simulink model "pendulum_model_PI"  (R2022b)
settings: Solver=VariableStepAuto  StartTime=0.0  StopTime=15  RelTol=1e-3
InitFcn:
  | % LRS TU KL %
  | % By Alen Turnwald %
  | % 09.01.2017 %
  | % clc
  | % close
  | 
  | %% g_q
  | % g_q = [1;0];
  | 
  | 
  | % if ~exist('mp','var')||~exist('mc','var')||~exist('L','var')||~exist('g','var')||~exist('d1','var')||~exist('d2','var')
  | % Model Paramter
  |     % warning(['(Some) Model Parameter are not defined!' ,10, '****  Setting the predefined parameter  ****'])
  |     % N = 2;
  |     % mc = 1.5;
  |     % mp = 0.5;
  |     % g = 9.82;
  |     % L = 1;
  | % Damping factors
  |     % d1 = 1e-2;
  |     % d2 = 1e-2;
  | % end
  | 
  | % if ~exist('x_0','var')
  | % Initial state
  |     % warning(['(Initial state "x_0" not defined or wrongly named!' ,10, '****  Setting x_0 = [0.1; 10 deg; 0; 0]  ****'])
  |     % x_0 = zeros(4,1);
  |     % x_0(1) = 0.1;
  |     % x_0(2) = 10*pi/180;
  | % end
  | 
  | % if ~exist('K_lqr','var')||~exist('Kd_lqr','var')
  | %    warning(['(No controller found!' ,10, '****   Applying a predefined controller  ****'])
  | %    K_lqr = [-14.1421  171.8846  -25.2787   54.7535];
  | % end
undefined symbols (not defined in the file or in its folder): A, B, b_pitching, b_rolling, disturbance, K_d_angle, K_i_pitch, K_p_pitch, period, pulse_width, stall_T, target_angle, x_0
libraries: slpidlib x1
settings Model: Creator=Jake  LastModifiedBy=Jake

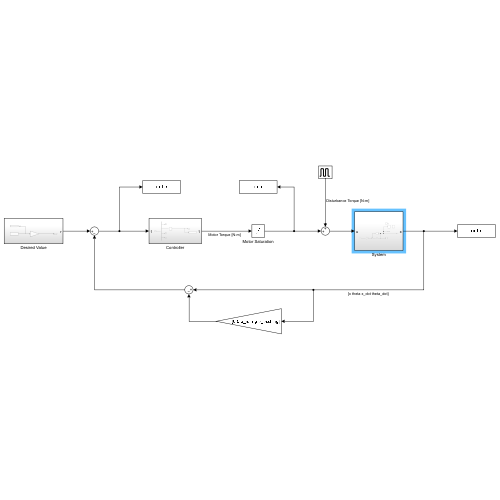
[thumbnail: Simulink's stored preview of the top-level diagram]
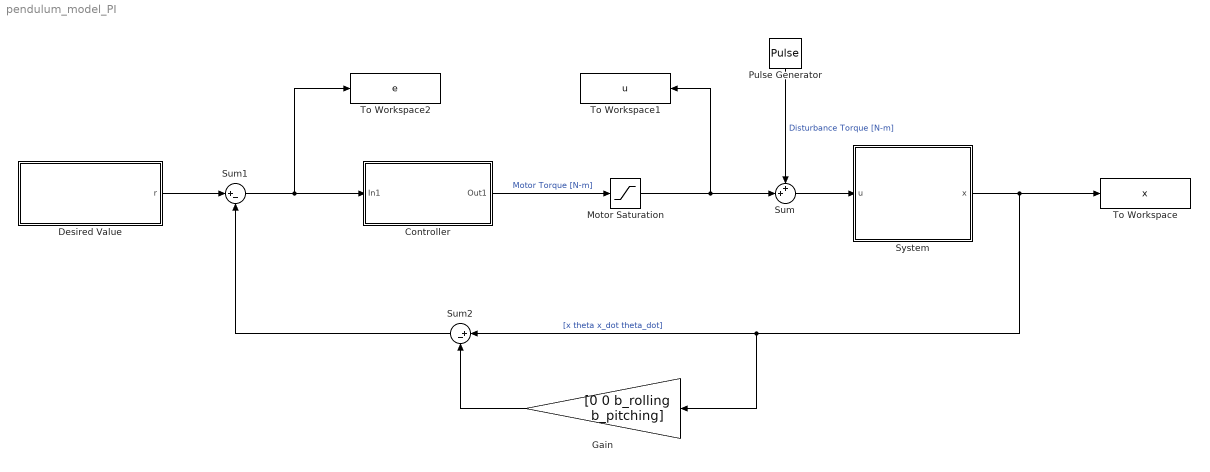
== system pendulum_model_PI ==
  Controller : Subsystem
  Desired Value : Subsystem
  Gain : Gain  Gain=[0 0 b_rolling b_pitching]
  Motor Saturation : Saturate  UpperLimit=stall_T  LowerLimit=-stall_T
  Pulse Generator : DiscretePulseGenerator  PulseType=Time based  Amplitude=disturbance  Period=period  PulseWidth=pulse_width
  Sum : Sum  Inputs=++|
  Sum1 : Sum  Inputs=|+-
  Sum2 : Sum  Inputs=|+-
  System : Subsystem
  To Workspace : ToWorkspace  VariableName=x  SampleTime=-1
  To Workspace1 : ToWorkspace  VariableName=u  SampleTime=-1
  To Workspace2 : ToWorkspace  VariableName=e  SampleTime=-1
  wires:
  Sum/1 -> System/1(u)
  Motor Saturation/1 -> To Workspace1/1, Sum/2
  Pulse Generator/1 -> Sum/1  "Disturbance Torque [N-m]"
  Desired Value/1(r) -> Sum1/1
  Controller/1(Out1) -> Motor Saturation/1  "Motor Torque [N-m]"
  Sum1/1 -> To Workspace2/1, Controller/1(In1)
  System/1(x) -> To Workspace/1, Sum2/1, Gain/1  "[x theta x_dot theta_dot]"
  Sum2/1 -> Sum1/2
  Gain/1 -> Sum2/2

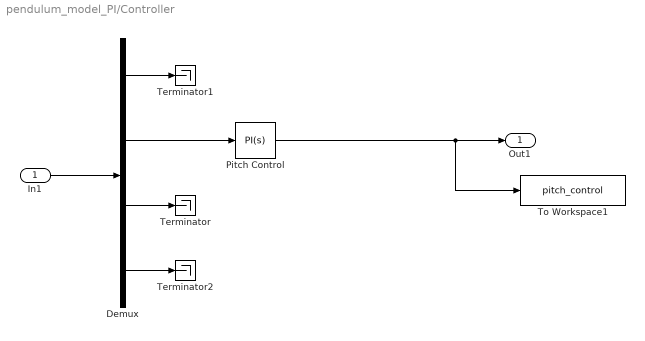
== system pendulum_model_PI/Controller ==
  In1 : Inport
  Demux : Demux
  Pitch Control : slpidlib/PID Controller  Controller=PI  Form=Parallel  TimeDomain=Continuous-time  UseExternalTs=off  SampleTime=-1  IntegratorMethod=Forward Euler  FilterMethod=Forward Euler  ControllerParametersSource=internal  P=K_p_pitch  I=K_i_pitch  UseKiTs=off  D=K_d_angle  N=45  UseFilter=on  TunerSelectOption=Transfer Function Based (PID Tuner App)  InitialConditionSource=internal  InitialConditionForIntegrator=0  InitialConditionForFilter=0  DifferentiatorICPrevScaledInput=0  ExternalReset=none  TrackingMode=off  Kt=1  LimitOutput=off  SatLimitsSource=internal  UpperSaturationLimit=inf  LowerSaturationLimit=-inf  LinearizeAsGain=on  AntiWindupMode=none  Kb=1  LimitIntegrator=off  UpperIntegratorSaturationLimit=inf  LowerIntegratorSaturationLimit=-inf  POutMin=[]  POutMax=[]  IOutMin=[]  IOutMax=[]  DOutMin=[]  DOutMax=[]  NOutMin=[]  NOutMax=[]  SumOutMin=[]  SumOutMax=[]  SaturationOutMin=[]  SaturationOutMax=[]  PParamMin=[]  PParamMax=[]  IParamMin=[]  IParamMax=[]  DParamMin=[]  DParamMax=[]  NParamMin=[]  NParamMax=[]  KbParamMin=[]  KbParamMax=[]  KtParamMin=[]  KtParamMax=[]  KbOutMin=[]  KbOutMax=[]  KtOutMin=[]  KtOutMax=[]  IntegratorOutMin=[]  IntegratorOutMax=[]  FilterOutMin=[]  FilterOutMax=[]  SumI1OutMin=[]  SumI1OutMax=[]  SumI2OutMin=[]  SumI2OutMax=[]  SumI3OutMin=[]  SumI3OutMax=[]  SumI4OutMin=[]  SumI4OutMax=[]  SumDOutMin=[]  SumDOutMax=[]  DifferentiatorOutMin=[]  DifferentiatorOutMax=[]  FilterDiffOutCoefMin=[]  FilterDiffOutCoefMax=[]  ReciprocalOutMin=[]  ReciprocalOutMax=[]  SumDenOutMin=[]  SumDenOutMax=[]  SumNumOutMin=[]  SumNumOutMax=[]  DivideOutMin=[]  DivideOutMax=[]  UdiffTsProdOutMin=[]  UdiffTsProdOutMax=[]  NTsProdOutMin=[]  NTsProdOutMax=[]  UintegralTsProdOutMin=[]  UintegralTsProdOutMax=[]  UngainTsProdOutMin=[]  UngainTsProdOutMax=[]  ClampingZeroOutDataTypeStr=Inherit: Inherit via back propagation  ClampingZeroOutMin=[]  ClampingZeroOutMax=[]  FilterDenConstantOutDataTypeStr=Inherit: Inherit via back propagation  FilterDenConstantOutMin=[]  FilterDenConstantOutMax=[]  PCopyOutDataTypeStr=Inherit: Inherit via back propagation  PCopyOutMin=[]  PCopyOutMax=[]  NCopyOutDataTypeStr=Inherit: Inherit via back propagation  NCopyOutMin=[]  NCopyOutMax=[]  IntegratorContinuousStateAttributes=''  IntegratorStateMustResolveToSignalObject=off  IntegratorRTWStateStorageClass=Auto  FilterContinuousStateAttributes=''  FilterStateMustResolveToSignalObject=off  FilterRTWStateStorageClass=Auto  ParallelPVariant=InternalParameters  IdealPVariant=Disabled  IVariant=InternalParameters  DVariant=Disabled  IntegratorVariant=Continuous  SatVariant=Disabled  AWVariant=Passthrough  PCopyVariant=Disabled  TRVariant=Disabled  FdbkBlocksVariant=Forward  IdealPFdbkVariant=Disabled  SatFdbkVariant=Disabled  DerivativeFilterVariant=Disabled  NVariant=Disabled  NCopyVariant=Disabled_SignalSpec  FilterICVariant=Disabled  IntegratorICVariant=InternalICs  ExternalResetVariant=Disabled  TRSumVariant=Passthrough  SumFdbkVariant=Disabled  SumVariant=Sum_PI  TsampFilterVariant=InternalTs  TsampNgainVariant=Passthrough  TsampIntegralVariant=Passthrough  ExternalSaturationOutDataTypeStr=Inherit: Same as second input
  Terminator : Terminator
  Terminator1 : Terminator
  Terminator2 : Terminator
  To Workspace1 : ToWorkspace  VariableName=pitch_control  SampleTime=-1
  Out1 : Outport
  wires:
  In1/1 -> Demux/1
  Pitch Control/1 -> To Workspace1/1, Out1/1
  Demux/4 -> Terminator2/1
  Demux/3 -> Terminator/1
  Demux/2 -> Pitch Control/1
  Demux/1 -> Terminator1/1

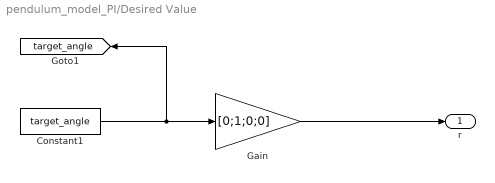
== system pendulum_model_PI/Desired Value ==
  Constant1 : Constant  Value=target_angle
  Gain : Gain  Gain=[0;1;0;0]
  r : Outport
  tag scope: target_angle=global
  wires:
  Constant1/1 -> Gain/1, [target_angle]
  Gain/1 -> r/1

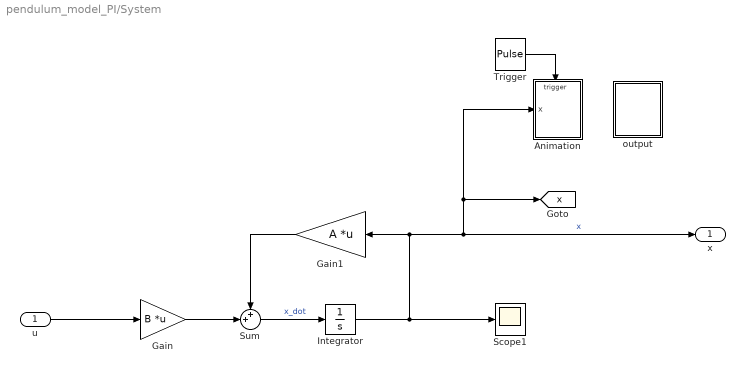
== system pendulum_model_PI/System ==
  u : Inport
  Animation : Subsystem
  Gain : Gain  Gain=B  Multiplication=Matrix(K*u)
  Gain1 : Gain  Gain=A  Multiplication=Matrix(K*u)
  Integrator : Integrator  InitialCondition=x_0
  Scope1 : Scope
  Sum : Sum  Inputs=++|
  Trigger : DiscretePulseGenerator  PulseType=Time based  Period=0.1  PulseWidth=50
  output : Subsystem
  x : Outport
  tag scope: x=global
  wires:
  u/1 -> Gain/1
  Sum/1 -> Integrator/1  "x_dot"
  Gain1/1 -> Sum/1
  Gain/1 -> Sum/2
  Integrator/1 -> Scope1/1, [x], Animation/1(x), x/1, Gain1/1  "x"
  Trigger/1 -> Animation/Trigger

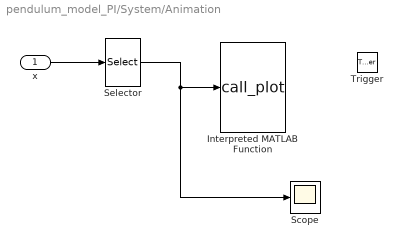
== system pendulum_model_PI/System/Animation ==
  x : Inport
  Trigger : TriggerPort  VariantControl=(inherit)  PortDimensions=1
  Interpreted MATLAB Function : MATLABFcn  MATLABFcn=call_plot  OutputDimensions=0
  Scope : Scope
  Selector : Selector  InputPortWidth=4  IndexOptions=Index vector (dialog)  Indices=[1:2]  OutputSizes=1
  wires:
  x/1 -> Selector/1
  Selector/1 -> Scope/1, Interpreted MATLAB Function/1

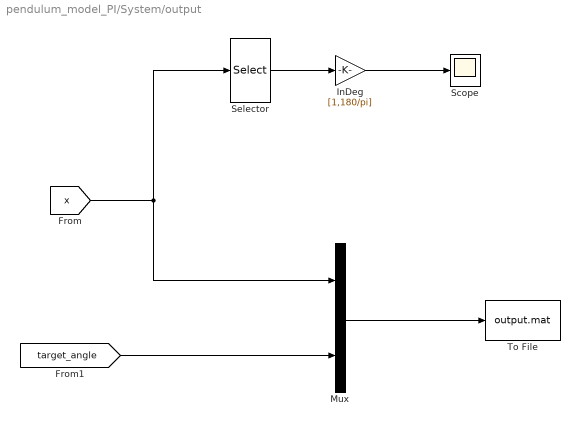
== system pendulum_model_PI/System/output ==
  InDeg : Gain  Gain=[1,180/pi]
  Mux : Mux  Inputs=2
  Scope : Scope
  Selector : Selector  InputPortWidth=4  IndexOptions=Index vector (dialog)  Indices=[1:2]  OutputSizes=1
  To File : ToFile  Filename=output.mat  MatrixName=out  SaveFormat=Timeseries
  wires:
  [x] -> Mux/1, Selector/1
  InDeg/1 -> Scope/1
  Selector/1 -> InDeg/1
  Mux/1 -> To File/1
  [target_angle] -> Mux/2
